simulink library "FAM_lab_scale"  (R2023b)
settings: Solver=VariableStepAuto  StartTime=0.0  StopTime=10.0  RelTol=1e-3
undefined symbols (not defined in the file): FAM_elasticity, FAM_unstretched_length, FAM_unstretched_radius, FAM_wall_thickness, fiber_angle_alpha
settings Model: Creator=cmmcguir  LastModifiedBy=Carson

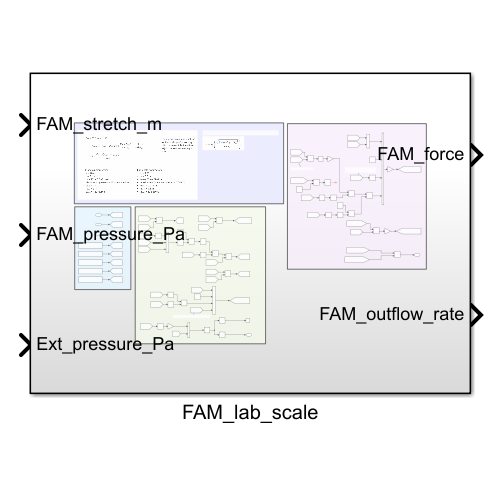
[thumbnail: Simulink's stored preview of the top-level diagram]
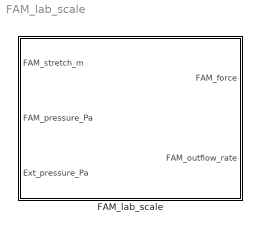
== system FAM_lab_scale ==
  FAM_lab_scale : Subsystem

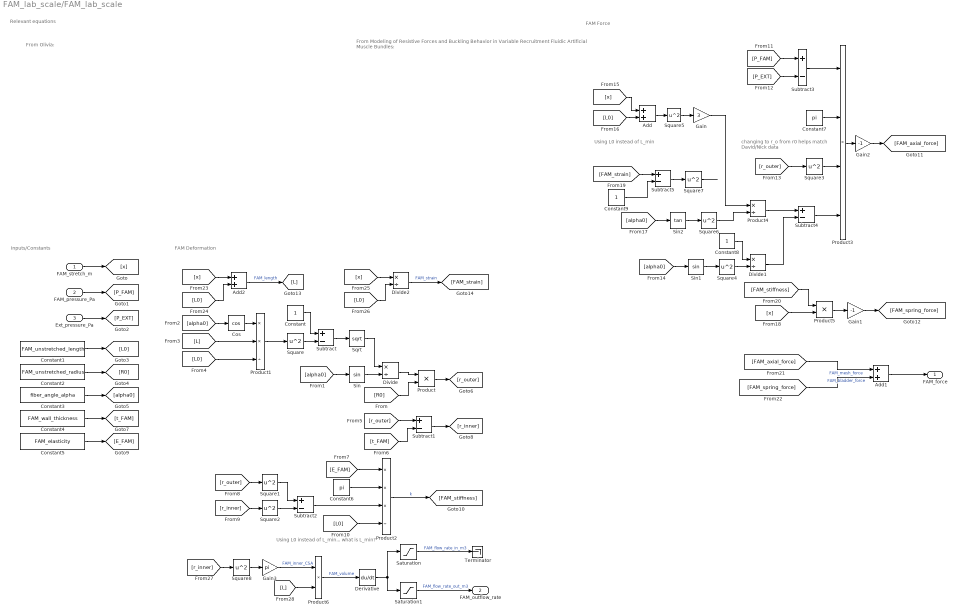
== system FAM_lab_scale/FAM_lab_scale ==
  note: FAM Force
  note: Using L0 instead of L_min
  note: changing to r_o from r0 helps match
      | David/Nick data
  note: FAM Deformation
  note: Inputs/Constants
  note: Relevant equations
  note: From Modeling of Resistive Forces and Buckling Behavior in Variable Recruitment Fluidic Artificial Muscle Bundles:
  note: From Olivia:
  note: Using L0 instead of L_min... what is L_min?
  FAM_stretch_m : Inport  Unit=m
  FAM_pressure_Pa : Inport  Port=2  Unit=Pa
  Ext_pressure_Pa : Inport  Port=3  Unit=Pa
  Add : Sum
  Add1 : Sum
  Add2 : Sum
  Constant : Constant
  Constant1 : Constant  Value=FAM_unstretched_length
  Constant2 : Constant  Value=FAM_unstretched_radius
  Constant3 : Constant  Value=fiber_angle_alpha
  Constant4 : Constant  Value=FAM_wall_thickness
  Constant5 : Constant  Value=FAM_elasticity
  Constant6 : Constant  Value=pi
  Constant7 : Constant  Value=pi
  Constant8 : Constant
  Constant9 : Constant
  Cos : Trigonometry  Operator=cos
  Derivative : Derivative
  Divide : Product  Inputs=*/
  Divide1 : Product  Inputs=*/
  Divide2 : Product  Inputs=*/
  Gain : Gain  Gain=3
  Gain1 : Gain  Gain=-1
  Gain2 : Gain  Gain=-1
  Gain3 : Gain  Gain=pi
  Product : Product
  Product1 : Product  Inputs=**/
  Product2 : Product  Inputs=***/
  Product3 : Product  Inputs=****
  Product4 : Product  Inputs=*/
  Product5 : Product
  Product6 : Product
  Saturation : Saturate  UpperLimit=inf  LowerLimit=0
  Saturation1 : Saturate  UpperLimit=0  LowerLimit=-inf
  Sin : Trigonometry
  Sin1 : Trigonometry
  Sin2 : Trigonometry  Operator=tan
  Sqrt : Sqrt
  Square{,1..8} (9 alike) : Math  Operator=square
  Subtract{,1..5} (6 alike) : Sum  Inputs=+-
  Terminator : Terminator
  FAM_force : Outport
  FAM_outflow_rate : Outport  Port=2
  wires:
  [x] -> Product5/2
  [E_FAM] -> Product2/1
  [FAM_axial_force] -> Add1/1  "FAM_mesh_force"
  [alpha0] -> Sin2/1
  Constant3/1 -> [alpha0]
  Gain/1 -> Product4/1
  [R0] -> Product/2
  Product2/1 -> [FAM_stiffness]  "k"
  [L0] -> Add/2
  [t_FAM] -> Subtract1/2
  Constant2/1 -> [R0]
  Ext_pressure_Pa/1 -> [P_EXT]
  [alpha0] -> Cos/1
  [FAM_stiffness] -> Product5/1
  Subtract2/1 -> Product2/3
  Product/1 -> [r_outer]
  [alpha0] -> Sin1/1
  Product5/1 -> Gain1/1
  Constant4/1 -> [t_FAM]
  Square6/1 -> Product4/2
  Cos/1 -> Product1/1
  Product3/1 -> Gain2/1
  FAM_pressure_Pa/1 -> [P_FAM]
  Subtract/1 -> Sqrt/1
  Constant7/1 -> Product3/2
  [FAM_spring_force] -> Add1/2  "FAM_bladder_force"
  Constant/1 -> Subtract/1
  [P_EXT] -> Subtract3/2
  [L0] -> Product2/4
  Add1/1 -> FAM_force/1
  Sin2/1 -> Square6/1
  [r_outer] -> Square1/1
  Product4/1 -> Subtract4/1
  Constant1/1 -> [L0]
  Square/1 -> Subtract/2
  Constant6/1 -> Product2/2
  FAM_stretch_m/1 -> [x]
  Divide1/1 -> Subtract4/2
  Subtract4/1 -> Product3/4
  Constant8/1 -> Divide1/1
  Divide/1 -> Product/1
  Sin1/1 -> Square4/1
  Subtract3/1 -> Product3/1
  Square3/1 -> Product3/3
  Square4/1 -> Divide1/2
  [r_outer] -> Subtract1/1
  [P_FAM] -> Subtract3/1
  Subtract1/1 -> [r_inner]
  [L0] -> Product1/3
  Sqrt/1 -> Divide/1
  [L] -> Product1/2
  Square1/1 -> Subtract2/1
  [x] -> Add/1
  Product1/1 -> Square/1
  Constant5/1 -> [E_FAM]
  [r_outer] -> Square3/1
  Square2/1 -> Subtract2/2
  Sin/1 -> Divide/2
  [alpha0] -> Sin/1
  [r_inner] -> Square2/1
  Square5/1 -> Gain/1
  Add/1 -> Square5/1
  [x] -> Add2/1
  [L0] -> Add2/2
  Add2/1 -> [L]  "FAM_length"
  Divide2/1 -> [FAM_strain]  "FAM_strain"
  [L0] -> Divide2/2
  [x] -> Divide2/1
  Gain1/1 -> [FAM_spring_force]
  [FAM_strain] -> Subtract5/1
  Constant9/1 -> Subtract5/2
  Subtract5/1 -> Square7/1
  Square7/1 -> ?
  Gain2/1 -> [FAM_axial_force]
  [r_inner] -> Square8/1
  Square8/1 -> Gain3/1
  Gain3/1 -> Product6/1  "FAM_inner_CSA"
  [L] -> Product6/2
  Product6/1 -> Derivative/1  "FAM_volume"
  Derivative/1 -> Saturation1/1, Saturation/1
  Saturation/1 -> Terminator/1  "FAM_flow_rate_in_m3"
  Saturation1/1 -> FAM_outflow_rate/1  "FAM_flow_rate_out_m3"
